simulink model "stereo_ibvs_core_backup_20260724_004703"  (R2025b)
settings: Solver=FixedStepDiscrete  StartTime=0.0  StopTime=inf  FixedStep=cfg.Ts  RelTol=1e-3
InitFcn:
  | cfgValid__=evalin('base','exist(''cfg'',''var'')==1 && isstruct(cfg) && all(isfield(cfg,{''Ts'',''robot'',''qInitial'',''zoomInitialSteps'',''cameraIntrinsicsStage1'',''rhoD'',''stereoBaseline'',''centerDesired'',''Kc'',''lambdaC'',''qMin'',''qMax'',''qLimitSoftMargin'',''qDotAlgorithmMax'',''stage1CalibrationReady''}))');if ~cfgValid__,modelFile__=get_param(bdroot,'FileName');modelDir__=fileparts(modelFile__);config1__=fullfile(modelDir__,'stereo_ibvs_config.m');config2__=fullfile(fileparts(modelDir__),'config','stereo_ibvs_config.m');if isfile(config1__),run(config1__);elseif isfile(config2__),run(config2__);else,error('StereoIBVS:ConfigNotFound','找不到stereo_ibvs_config.m。');end;end;clear cfgValid__ modelFile__ modelDir__ config1__ config2__
undefined symbols (not defined in the file): cfg, cfg_baseline, cfg_ekfCovarianceJitter, cfg_ekfInitializationMode, cfg_ekfP0, cfg_ekfRequireNewMeasurement, cfg_ekfSConditionMin, cfg_ekfX0, cfg_focalLength0Mm, cfg_fr3Axis, cfg_fr3Joint8OriginRPY, cfg_fr3Joint8OriginXYZ, cfg_fr3OriginRPY, cfg_fr3OriginXYZ, cfg_numericalEpsilon, cfg_pixelNoiseStd, cfg_q0, cfg_rhoMax, cfg_rhoMin, cfg_sigmaJerk, cfg_T_CL_CR, cfg_T_link8_CL, cfg_T_W_B, cfg_Ts, cfg_visibilityZMin
(part 4 of 4)

== matlab function stereo_ibvs_core_backup_20260724_004703/03_Feature_Processing/Normalize and Validate Features ==
  data: pixelMeasurement input; normalizedFeatureMeasured output; scaleMeasuredRaw input; fxMeasuredPx input; fyMeasuredPx input; validLeft input; validRight input; visionMeasurementNew input; resetSafe input; cfg_numericalEpsilon input; cfg_cxL input; cfg_cyL input; cfg_cxR input; cfg_cyR input; cfg_baseline input; cfg_disparityMin input; cfg_rhoMin input; cfg_rhoMax input; cfg_rightReacquireValidSamples input; cLMeasured output; cRMeasured output; scaleMeasured output; zMeasured output; xLeftMeasured output; yLeftMeasured output; xRightMeasured output; disparityNormalized output; rhoMeasured output; validDisparity output; stereoMeasurementEnable output; validStereoQualified output; rightReacquireActive output; rightReacquireCount output; uRightMeasured output
function [ ...
    normalizedFeatureMeasured, ...
    cLMeasured, ...
    cRMeasured, ...
    scaleMeasured, ...
    zMeasured, ...
    xLeftMeasured, ...
    yLeftMeasured, ...
    xRightMeasured, ...
    disparityNormalized, ...
    rhoMeasured, ...
    validDisparity, ...
    stereoMeasurementEnable, ...
    validStereoQualified, ...
    rightReacquireActive, ...
    rightReacquireCount, ...
    uRightMeasured] = fcn( ...
    pixelMeasurement, ...
    scaleMeasuredRaw, ...
    fxMeasuredPx, ...
    fyMeasuredPx, ...
    validLeft, ...
    validRight, ...
    visionMeasurementNew, ...
    resetSafe, ...
    cfg_numericalEpsilon, ...
    cfg_cxL, ...
    cfg_cyL, ...
    cfg_cxR, ...
    cfg_cyR, ...
    cfg_baseline, ...
    cfg_disparityMin, ...
    cfg_rhoMin, ...
    cfg_rhoMax, ...
    cfg_rightReacquireValidSamples)
%#codegen
% V2实机视觉测量提取与双目有效性管理。
% cfg_* 均由外部 Constant 块输入，不再登记为 MATLAB Function Parameter。

%% 固定尺寸输出
normalizedFeatureMeasured = zeros(4,1);
cLMeasured = zeros(2,1);
cRMeasured = zeros(2,1);
scaleMeasured = zeros(2,1);
zMeasured = zeros(3,1);

xLeftMeasured = 0;
yLeftMeasured = 0;
xRightMeasured = 0;
disparityNormalized = 0;
rhoMeasured = 0;

validDisparity = 0;
stereoMeasurementEnable = 0;
validStereoQualified = 0;
rightReacquireActive = 0;
rightReacquireCount = 0;
uRightMeasured = 0;

%% 右相机重捕获状态
persistent consecutiveValid reacquire

if isempty(consecutiveValid)
    consecutiveValid = 0.0;
    reacquire = 1.0;
end

%% 输入整理
pixels = reshape(pixelMeasurement,4,1);
scales = reshape(scaleMeasuredRaw,2,1);
fx = reshape(fxMeasuredPx,2,1);
fy = reshape(fyMeasuredPx,2,1);

leftValidFlag = ...
    isfinite(validLeft) && validLeft > 0.5;
rightValidFlag = ...
    isfinite(validRight) && validRight > 0.5;
newMeasurement = ...
    isfinite(visionMeasurementNew) && visionMeasurementNew > 0.5;
resetRequested = ...
    isfinite(resetSafe) && resetSafe > 0.5;

parameterFinite = all(isfinite([ ...
    cfg_numericalEpsilon
    cfg_cxL
    cfg_cyL
    cfg_cxR
    cfg_cyR
    cfg_baseline
    cfg_disparityMin
    cfg_rhoMin
    cfg_rhoMax
    cfg_rightReacquireValidSamples]));

parameterValid = ...
    parameterFinite && ...
    cfg_numericalEpsilon > 0 && ...
    cfg_baseline > cfg_numericalEpsilon && ...
    cfg_disparityMin >= 0 && ...
    cfg_rhoMin > 0 && ...
    cfg_rhoMax >= cfg_rhoMin && ...
    cfg_rightReacquireValidSamples >= 1;

reacquireRequired = 1.0;
if parameterValid
    reacquireRequired = max( ...
        1.0, ...
        floor(cfg_rightReacquireValidSamples));
end

geometryInputFinite = ...
    all(isfinite(pixels)) && ...
    all(isfinite(fx)) && ...
    all(isfinite(fy)) && ...
    parameterValid;

leftIntrinsicsValid = ...
    geometryInputFinite && ...
    fx(1) > cfg_numericalEpsilon && ...
    fy(1) > cfg_numericalEpsilon;

rightIntrinsicsValid = ...
    geometryInputFinite && ...
    fx(2) > cfg_numericalEpsilon && ...
    fy(2) > cfg_numericalEpsilon;

leftFeatureValid = ...
    leftValidFlag && leftIntrinsicsValid;
rightFeatureValid = ...
    rightValidFlag && rightIntrinsicsValid;

%% 像素坐标归一化
if leftFeatureValid
    cLMeasured = [ ...
        (pixels(1) - cfg_cxL) / fx(1)
        (pixels(2) - cfg_cyL) / fy(1)];
end

if rightFeatureValid
    cRMeasured = [ ...
        (pixels(3) - cfg_cxR) / fx(2)
        (pixels(4) - cfg_cyR) / fy(2)];

    % 只有右相机测量有效时才输出右相机像素位置。
    uRightMeasured = pixels(3);
end

% Scale无效时仅将对应Scale置零，不影响中心和双目几何计算。
if leftFeatureValid && ...
        isfinite(scales(1)) && scales(1) > 0
    scaleMeasured(1) = scales(1);
end

if rightFeatureValid && ...
        isfinite(scales(2)) && scales(2) > 0
    scaleMeasured(2) = scales(2);
end

normalizedFeatureMeasured = [cLMeasured; cRMeasured];

xLeftMeasured = cLMeasured(1);
yLeftMeasured = cLMeasured(2);
xRightMeasured = cRMeasured(1);

%% 双目视差与逆深度测量
if leftFeatureValid && rightFeatureValid
    disparityNormalized = ...
        xLeftMeasured - xRightMeasured;

    candidateRho = ...
        disparityNormalized / cfg_baseline;

    validDisparity = double( ...
        isfinite(candidateRho) && ...
        disparityNormalized > cfg_disparityMin && ...
        candidateRho >= cfg_rhoMin && ...
        candidateRho <= cfg_rhoMax);

    if validDisparity > 0.5
        rhoMeasured = candidateRho;
    end
end

zMeasured = [ ...
    xLeftMeasured
    yLeftMeasured
    rhoMeasured];

%% 完整有限值保护
measurementOutputsFinite = ...
    all(isfinite(normalizedFeatureMeasured)) && ...
    all(isfinite(cLMeasured)) && ...
    all(isfinite(cRMeasured)) && ...
    all(isfinite(scaleMeasured)) && ...
    all(isfinite(zMeasured)) && ...
    isfinite(xLeftMeasured) && ...
    isfinite(yLeftMeasured) && ...
    isfinite(xRightMeasured) && ...
    isfinite(disparityNormalized) && ...
    isfinite(rhoMeasured) && ...
    isfinite(validDisparity) && ...
    isfinite(uRightMeasured);

if ~measurementOutputsFinite
    normalizedFeatureMeasured = zeros(4,1);
    cLMeasured = zeros(2,1);
    cRMeasured = zeros(2,1);
    scaleMeasured = zeros(2,1);
    zMeasured = zeros(3,1);

    xLeftMeasured = 0;
    yLeftMeasured = 0;
    xRightMeasured = 0;
    disparityNormalized = 0;
    rhoMeasured = 0;
    validDisparity = 0;
    uRightMeasured = 0;
end

%% 双目资格与右相机重捕获管理
rawStereoValid = ...
    measurementOutputsFinite && ...
    leftFeatureValid && ...
    rightFeatureValid && ...
    validDisparity > 0.5;

if resetRequested
    consecutiveValid = 0.0;
    reacquire = 1.0;

elseif newMeasurement
    if rawStereoValid
        consecutiveValid = min( ...
            consecutiveValid + 1.0, ...
            reacquireRequired);
    else
        consecutiveValid = 0.0;
    end

    if ~rawStereoValid
        reacquire = 1.0;
    elseif consecutiveValid >= reacquireRequired
        reacquire = 0.0;
    end
end

validStereoQualified = double( ...
    rawStereoValid && ...
    consecutiveValid >= reacquireRequired);

% 每个新视觉测量最多触发一次EKF校正。
stereoMeasurementEnable = double( ...
    newMeasurement && ...
    validStereoQualified > 0.5 && ...
    ~resetRequested);

rightReacquireActive = double( ...
    leftFeatureValid && ...
    reacquire > 0.5);

rightReacquireCount = consecutiveValid;
end
